simulink model "Project2_Trial"  (R2014a)
settings: Solver=ode45  StartTime=0.0  StopTime=100  RelTol=1e-3
libraries: simulink x1
settings Model: Creator=dzr3qn  LastModifiedBy=dzr3qn

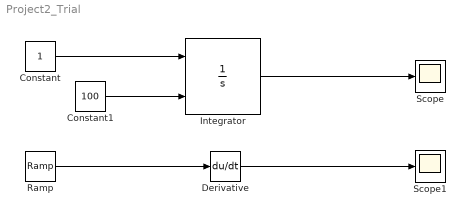
== system Project2_Trial ==
  Constant : Constant
  Constant1 : Constant  Value=100
  Derivative : Derivative
  Integrator : Integrator  InitialConditionSource=external
  Ramp : simulink/Sources/Ramp  slope=1  start=0  X0=0
  Scope : Scope
  Scope1 : Scope
  wires:
  Constant/1 -> Integrator/1
  Integrator/1 -> Scope/1
  Derivative/1 -> Scope1/1
  Ramp/1 -> Derivative/1
  Constant1/1 -> Integrator/2
